simulink model "ex01_object_tracking_static_demo"  (Simulink 7.3)
settings: Solver=FixedStepDiscrete  StartTime=0.0  StopTime=.01  FixedStep=.02  RelTol=1e-3
InitFcn:
  | hsize = 20;
  | sigma = 10;
  | gaus_filt = fspecial('gaussian',hsize , sigma);
undefined symbols (not defined in the file): gray
libraries: vipsnks x6, viptextngfix x2, vipsrcs x2, vipfilter x1
settings Model: Creator=Krisada  LastModifiedBy=Krisada

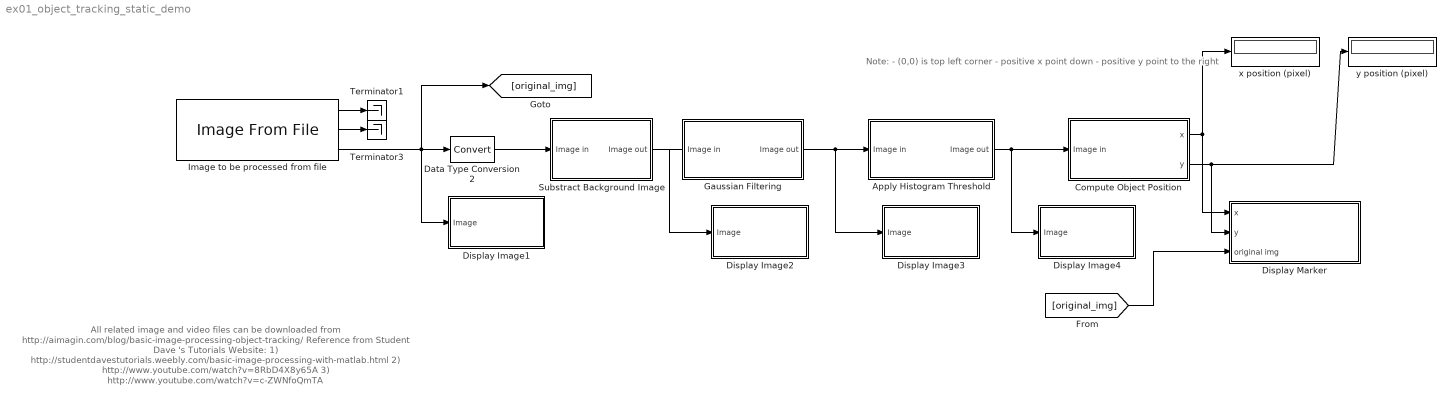
== system ex01_object_tracking_static_demo ==
  note: All related image and video files can be downloaded from http://aimagin.com/blog/basic-image-processing-object-tracking/
      | Reference from Student Dave 's Tutorials Website:
      | 1) http://studentdavestutorials.weebly.com/basic-image-processing-with-matlab.html
      | 2) http://www.youtube.com/watch?v=8RbD4X8y65A
      | 3) http://www.youtube.com/watch?v=c-ZWNfoQmTA
  note: Note:
      | - (0,0) is top left corner
      | - positive x point down
      | - positive y point to the right
  Apply Histogram Threshold : Subsystem
  Compute Object Position : Subsystem
  Data Type Conversion2 : DataTypeConversion  OutDataType=fixdt(1, 16)  OutScaling=2^0
  Display Image1 : Subsystem
  Display Image2 : Subsystem
  Display Image3 : Subsystem
  Display Image4 : Subsystem
  Display Marker : Subsystem
  Gaussian Filtering : Subsystem
  Image to be processed from file : vipsrcs/Image From File  Tag=vipblks_nd  DialogController=vipDDGCreate  DialogControllerArgs=DataTag13  SystemSampleTime=-1  FileName=D:\waijung\trunk\waijung\targets\stm32f4_target\stm32f4\demo\image_object_tracking_demo\hexbug_vid0155.png  imagePorts=Separate color signals  Ts=inf  ImageDataType=Inherit from input image  Signed=on  WordLength=16  sdImageDataType=uint(8)  FractionLengthMode=User-defined  FractionLength=15  OutPortLabels=R|G|B
  Substract Background Image : Subsystem
  Terminator1 : Terminator
  Terminator3 : Terminator
  x position (pixel) : Display
  y position (pixel) : Display
  wires:
  Gaussian Filtering/1(Image out) -> Apply Histogram Threshold/1(Image in), Display Image3/1(Image)
  Substract Background Image/1(Image out) -> Gaussian Filtering/1(Image in), Display Image2/1(Image)
  Apply Histogram Threshold/1(Image out) -> Display Image4/1(Image), Compute Object Position/1(Image in)
  Image to be processed from file/3 -> [original_img], Data Type Conversion2/1, Display Image1/1(Image)
  Image to be processed from file/1 -> Terminator1/1
  Image to be processed from file/2 -> Terminator3/1
  Data Type Conversion2/1 -> Substract Background Image/1(Image in)
  Compute Object Position/1(x) -> x position (pixel)/1, Display Marker/1(x)
  Compute Object Position/2(y) -> y position (pixel)/1, Display Marker/2(y)
  [original_img] -> Display Marker/3(original img)

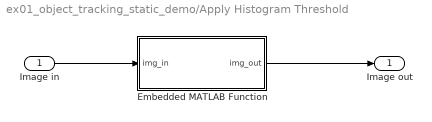
== system ex01_object_tracking_static_demo/Apply Histogram Threshold ==
  Image in : Inport
  Embedded MATLAB Function : Stateflow chart
  Image out : Outport
  wires:
  Image in/1 -> Embedded MATLAB Function/1(img_in)
  Embedded MATLAB Function/1(img_out) -> Image out/1

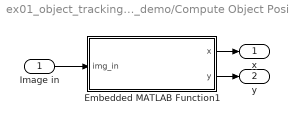
== system ex01_object_tracking_static_demo/Compute Object Position ==
  Image in : Inport
  Embedded MATLAB Function1 : Stateflow chart
  x : Outport
  y : Outport  Port=2
  wires:
  Image in/1 -> Embedded MATLAB Function1/1(img_in)
  Embedded MATLAB Function1/1(x) -> x/1
  Embedded MATLAB Function1/2(y) -> y/1

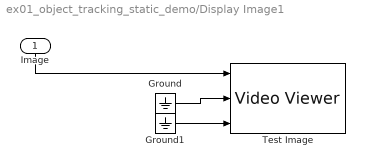
== system ex01_object_tracking_static_demo/Display Image1 ==
  Image : Inport
  Ground : Ground
  Ground1 : Ground
  Test Image : vipsnks/Video Viewer  DialogControllerArgs=DataTag1  inputType=Obsolete7b  imagePorts=Separate color signals  useColorMap=off  colormapValue=gray(256)  specRange=off  minInputVal=0  maxInputVal=255  FigPos=[1056 516 410 398]  AxisZoom=on  trueSizedOnce=off  OpenAtMdlStart=on
  wires:
  Image/1 -> Test Image/1
  Ground1/1 -> Test Image/3
  Ground/1 -> Test Image/2

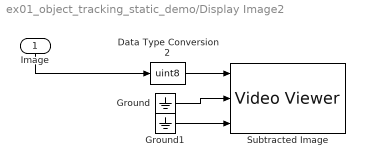
== system ex01_object_tracking_static_demo/Display Image2 ==
  Image : Inport
  Data Type Conversion2 : DataTypeConversion  OutDataTypeMode=uint8  OutDataType=fixdt(1, 16)  OutScaling=2^0  OutDataTypeStr=uint8
  Ground : Ground
  Ground1 : Ground
  Subtracted Image : vipsnks/Video Viewer  DialogControllerArgs=DataTag3  inputType=Obsolete7b  imagePorts=Separate color signals  useColorMap=off  colormapValue=gray(256)  specRange=off  minInputVal=0  maxInputVal=255  FigPos=[618 1033 410 398]  AxisZoom=on  trueSizedOnce=off  OpenAtMdlStart=on
  wires:
  Data Type Conversion2/1 -> Subtracted Image/1
  Ground/1 -> Subtracted Image/2
  Ground1/1 -> Subtracted Image/3
  Image/1 -> Data Type Conversion2/1

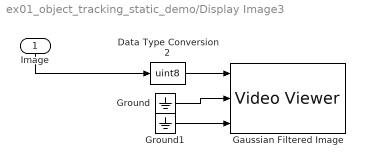
== system ex01_object_tracking_static_demo/Display Image3 ==
  Image : Inport
  Data Type Conversion2 : DataTypeConversion  OutDataTypeMode=uint8  OutDataType=fixdt(1, 16)  OutScaling=2^0  OutDataTypeStr=uint8
  Gaussian Filtered Image : vipsnks/Video Viewer  DialogControllerArgs=DataTag5  inputType=Obsolete7b  imagePorts=Separate color signals  useColorMap=off  colormapValue=gray(256)  specRange=off  minInputVal=0  maxInputVal=255  FigPos=[622 516 410 398]  AxisZoom=on  trueSizedOnce=off  OpenAtMdlStart=on
  Ground : Ground
  Ground1 : Ground
  wires:
  Data Type Conversion2/1 -> Gaussian Filtered Image/1
  Ground/1 -> Gaussian Filtered Image/2
  Ground1/1 -> Gaussian Filtered Image/3
  Image/1 -> Data Type Conversion2/1

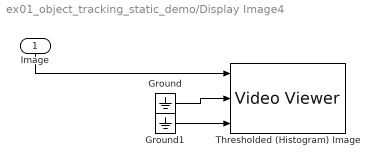
== system ex01_object_tracking_static_demo/Display Image4 ==
  Image : Inport
  Ground : Ground
  Ground1 : Ground
  Thresholded (Histogram) Image : vipsnks/Video Viewer  DialogControllerArgs=DataTag7  inputType=Obsolete7b  imagePorts=Separate color signals  useColorMap=off  colormapValue=gray(256)  specRange=off  minInputVal=0  maxInputVal=255  FigPos=[1492 513 410 398]  AxisZoom=on  trueSizedOnce=off  OpenAtMdlStart=on
  wires:
  Image/1 -> Thresholded (Histogram) Image/1
  Ground1/1 -> Thresholded (Histogram) Image/3
  Ground/1 -> Thresholded (Histogram) Image/2

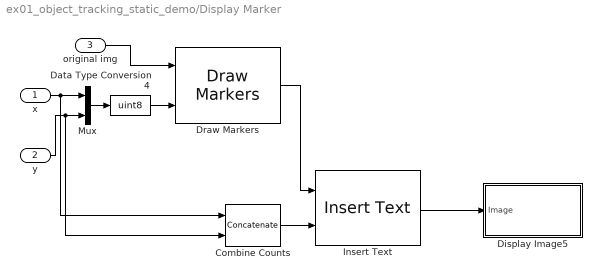
== system ex01_object_tracking_static_demo/Display Marker ==
  x : Inport
  y : Inport  Port=2
  original img : Inport  Port=3
  Combine Counts : Concatenate  Mode=Multidimensional array  ConcatenateDimension=2
  Data Type Conversion4 : DataTypeConversion  OutDataTypeMode=uint8  OutDataType=fixdt(1, 16)  OutScaling=2^0  OutDataTypeStr=uint8
  Display Image5 : Subsystem
  Draw Markers : viptextngfix/Draw Markers  DialogController=vipDDGCreate  DialogControllerArgs=DataTag10  shape=Square  size=5  fill=on  fillClrSource=Specify via dialog  display=White  intensity=200  color=1.5  opacity=0.6  viewport=Entire image  antialiasing=off  inType=Obsolete  imagePorts=One multidimensional signal  prodOutputMode=Binary point scaling  prodOutputWordLength=32  prodOutputFracLength=14  memoryMode=Specify word length  memoryWordLength=16  memoryFracLength=14  roundingMode=Floor  overflowMode=off
  Insert Text : viptextngfix/Insert Text  DialogController=vipDDGCreate  DialogControllerArgs=DataTag11  inputType=Obsolete  theText='x: %3.2f, y: %3.2f'  fontFace=LucidaSansRegular  dummyVar1=0  blockFontSize=12  antiAliased=on  getTextLocFrom=Specify via dialog  textLoc=[20 150]  getTextColorFrom=Specify via dialog  textColor=[0 255 0]  getTextIntensityFrom=Specify via dialog  textIntensity=0  getTextOpacityFrom=Specify via dialog  textOpacity=1.0  dummyVar2=0  dummyVar3=0  dummyVar4=0  imagePorts=One multidimensional signal  isInputTransposed=off
  Mux : Mux  Inputs=2
  wires:
  Mux/1 -> Data Type Conversion4/1
  Data Type Conversion4/1 -> Draw Markers/2
  original img/1 -> Draw Markers/1
  x/1 -> Mux/1, Combine Counts/1
  y/1 -> Mux/2, Combine Counts/2
  Draw Markers/1 -> Insert Text/1
  Combine Counts/1 -> Insert Text/2
  Insert Text/1 -> Display Image5/1(Image)

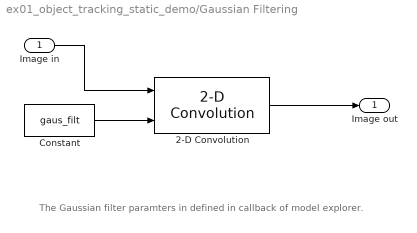
== system ex01_object_tracking_static_demo/Gaussian Filtering ==
  note: The Gaussian filter paramters in defined in callback of model explorer.
  Image in : Inport
  2-D Convolution : vipfilter/2-D Convolution  DialogController=vipDDGCreate  DialogControllerArgs=DataTag12  outSize=Same as input port I1  normalize=off  outputMode=Binary point scaling  outputWordLength=32  outputFracLength=12  prodOutputMode=Binary point scaling  prodOutputWordLength=32  prodOutputFracLength=10  roundingMode=Floor  overflowMode=off
  Constant : Constant  Value=gaus_filt  VectorParams1D=off  OutDataType=fixdt(1, 16)  OutScaling=2^0
  Image out : Outport
  wires:
  Constant/1 -> 2-D Convolution/2
  Image in/1 -> 2-D Convolution/1
  2-D Convolution/1 -> Image out/1

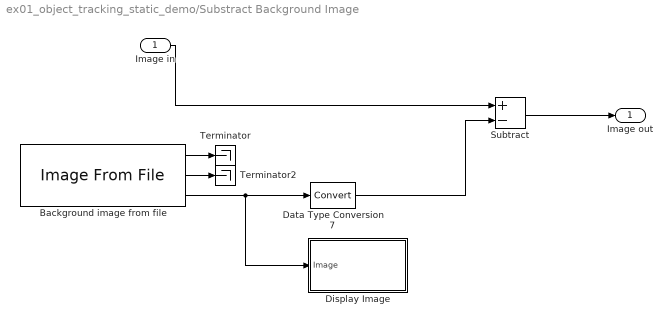
== system ex01_object_tracking_static_demo/Substract Background Image ==
  Image in : Inport
  Background image from file : vipsrcs/Image From File  Tag=vipblks_nd  DialogController=vipDDGCreate  DialogControllerArgs=DataTag14  SystemSampleTime=-1  FileName=D:\waijung\trunk\waijung\targets\stm32f4_target\stm32f4\demo\image_object_tracking_demo\hexbug_vid0000.png  imagePorts=Separate color signals  Ts=inf  ImageDataType=Inherit from input image  Signed=on  WordLength=16  sdImageDataType=uint(8)  FractionLengthMode=User-defined  FractionLength=15  OutPortLabels=R|G|B
  Data Type Conversion7 : DataTypeConversion  OutDataType=fixdt(1, 16)  OutScaling=2^0
  Display Image : Subsystem
  Subtract : Sum  Inputs=+-  OutDataType=fixdt(1, 16)  OutScaling=2^-10  RndMeth=Nearest
  Terminator : Terminator
  Terminator2 : Terminator
  Image out : Outport
  wires:
  Background image from file/3 -> Data Type Conversion7/1, Display Image/1(Image)
  Data Type Conversion7/1 -> Subtract/2
  Background image from file/1 -> Terminator/1
  Background image from file/2 -> Terminator2/1
  Image in/1 -> Subtract/1
  Subtract/1 -> Image out/1

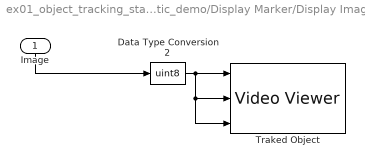
== system ex01_object_tracking_static_demo/Display Marker/Display Image5 ==
  Image : Inport
  Data Type Conversion2 : DataTypeConversion  OutDataTypeMode=uint8  OutDataType=fixdt(1, 16)  OutScaling=2^0  OutDataTypeStr=uint8
  Traked Object : vipsnks/Video Viewer  DialogControllerArgs=DataTag9  inputType=Obsolete7b  imagePorts=Separate color signals  useColorMap=off  colormapValue=gray(256)  specRange=off  minInputVal=0  maxInputVal=255  FigPos=[1056 1035 410 398]  AxisZoom=on  trueSizedOnce=off  OpenAtMdlStart=on
  wires:
  Data Type Conversion2/1 -> Traked Object/1, Traked Object/2, Traked Object/3
  Image/1 -> Data Type Conversion2/1

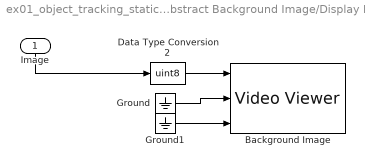
== system ex01_object_tracking_static_demo/Substract Background Image/Display Image ==
  Image : Inport
  Background Image : vipsnks/Video Viewer  DialogControllerArgs=DataTag16  inputType=Obsolete7b  imagePorts=Separate color signals  useColorMap=off  colormapValue=gray(256)  specRange=off  minInputVal=0  maxInputVal=255  FigPos=[1492 1034 410 398]  AxisZoom=on  trueSizedOnce=off  OpenAtMdlStart=on
  Data Type Conversion2 : DataTypeConversion  OutDataTypeMode=uint8  OutDataType=fixdt(1, 16)  OutScaling=2^0  OutDataTypeStr=uint8
  Ground : Ground
  Ground1 : Ground
  wires:
  Data Type Conversion2/1 -> Background Image/1
  Ground/1 -> Background Image/2
  Ground1/1 -> Background Image/3
  Image/1 -> Data Type Conversion2/1

== matlab function Compute Object Position/Embedded MATLAB Function1 ==
  data: img_in input double; x output double; y output double
function [x,y] = fcn(img_in)
	%#eml
	
	% size 352, 288
	sumx = 0;
	sumx_cnt = 0;
	for j = 1:352
		for i = 1:288
			if (img_in(i,j) ~= 0)
				sumx = sumx + i;
				sumx_cnt = sumx_cnt + 1;
			end
		end
	end
	if (sumx ~= 0)
		x = sumx/sumx_cnt;
	else
		x = 200;
	end
	
	sumy = 0;
	sumy_cnt = 0;
	for i = 1:288
		for j = 1:352
			if (img_in(i,j) ~= 0)
				sumy = sumy + j;
				sumy_cnt = sumy_cnt + 1;
			end
		end
	end
	if (sumy ~= 0)
		y = sumy/sumy_cnt;
	else
		y = 200;
	end

== matlab function Apply Histogram Threshold/Embedded MATLAB Function ==
  data: img_in input double; img_out output double
function img_out = fcn(img_in)
	%#eml
	
	img_out = (img_in < -20);
